simulink model "alfa147gta"  (R2013a)
settings: Solver=ode45  StartTime=0.0  StopTime=10.0  RelTol=1e-3
PreLoadFcn:
  | load('alfa147gta.mat')
undefined symbols (not defined in the file): EngineRPM, EngineTRQ, FinalRatio, GearRatio, Kdrag, Mass, WheelRadius
settings Model: Creator=luca  LastModifiedBy=luca

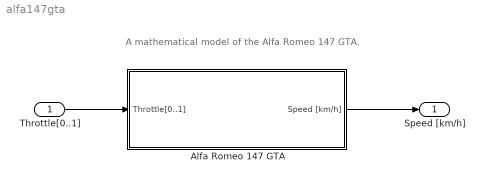
== system alfa147gta ==
  note: A mathematical model of the Alfa Romeo 147 GTA.
  Throttle[0..1] : Inport
  Alfa Romeo 147 GTA : Subsystem
  Speed [km/h] : Outport
  wires:
  Throttle[0..1]/1 -> Alfa Romeo 147 GTA/1(Throttle[0..1])
  Alfa Romeo 147 GTA/1(Speed [km/h]) -> Speed [km/h]/1

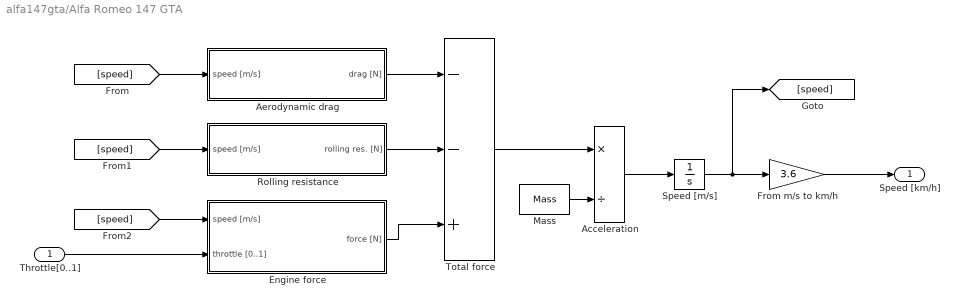
== system alfa147gta/Alfa Romeo 147 GTA ==
  Throttle[0..1] : Inport
  Acceleration : Product  Inputs=*/
  Aerodynamic drag : Subsystem
  Engine force : Subsystem
  From m/s to km/h : Gain  Gain=3.6
  Mass : Constant  Value=Mass
  Rolling resistance : Subsystem
  Speed [m/s] : Integrator
  Total force : Sum  Inputs=--+
  Speed [km/h] : Outport
  wires:
  Engine force/1(force [N]) -> Total force/3
  Rolling resistance/1(rolling res. [N]) -> Total force/2
  Aerodynamic drag/1(drag [N]) -> Total force/1
  Total force/1 -> Acceleration/1
  Mass/1 -> Acceleration/2
  Acceleration/1 -> Speed [m/s]/1
  Speed [m/s]/1 -> [speed], From m/s to km/h/1
  From m/s to km/h/1 -> Speed [km/h]/1
  [speed] -> Aerodynamic drag/1(speed [m/s])
  [speed] -> Rolling resistance/1(speed [m/s])
  Throttle[0..1]/1 -> Engine force/2(throttle [0..1])
  [speed] -> Engine force/1(speed [m/s])

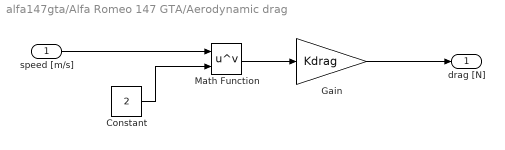
== system alfa147gta/Alfa Romeo 147 GTA/Aerodynamic drag ==
  speed [m/s] : Inport
  Constant : Constant  Value=2
  Gain : Gain  Gain=Kdrag
  Math Function : Math  Operator=pow  SaturateOnIntegerOverflow=on
  drag [N] : Outport
  wires:
  speed [m/s]/1 -> Math Function/1
  Constant/1 -> Math Function/2
  Math Function/1 -> Gain/1
  Gain/1 -> drag [N]/1

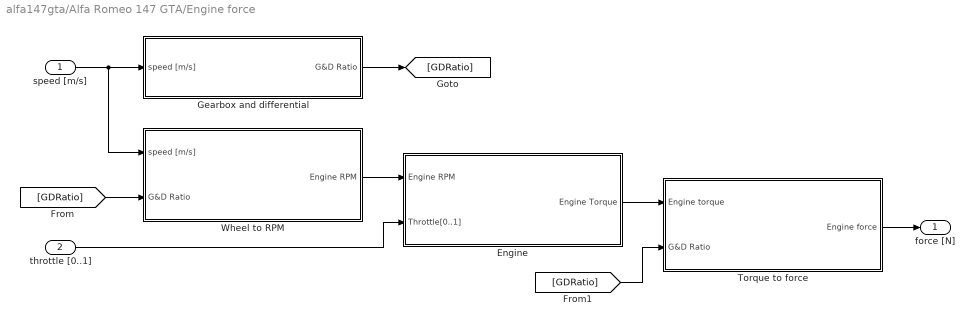
== system alfa147gta/Alfa Romeo 147 GTA/Engine force ==
  speed [m/s] : Inport
  throttle [0..1] : Inport  Port=2
  Engine : Subsystem
  Gearbox and differential : Subsystem
  Torque to force : Subsystem
  Wheel to RPM : Subsystem
  force [N] : Outport
  wires:
  Wheel to RPM/1(Engine RPM) -> Engine/1(Engine RPM)
  throttle [0..1]/1 -> Engine/2(Throttle[0..1])
  speed [m/s]/1 -> Gearbox and differential/1(speed [m/s]), Wheel to RPM/1(speed [m/s])
  Engine/1(Engine Torque) -> Torque to force/1(Engine torque)
  Torque to force/1(Engine force) -> force [N]/1
  Gearbox and differential/1(G&D Ratio) -> [GDRatio]
  [GDRatio] -> Wheel to RPM/2(G&D Ratio)
  [GDRatio] -> Torque to force/2(G&D Ratio)

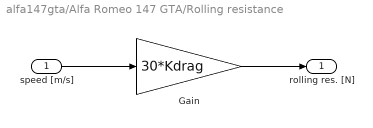
== system alfa147gta/Alfa Romeo 147 GTA/Rolling resistance ==
  speed [m/s] : Inport
  Gain : Gain  Gain=30*Kdrag
  rolling res. [N] : Outport
  wires:
  speed [m/s]/1 -> Gain/1
  Gain/1 -> rolling res. [N]/1

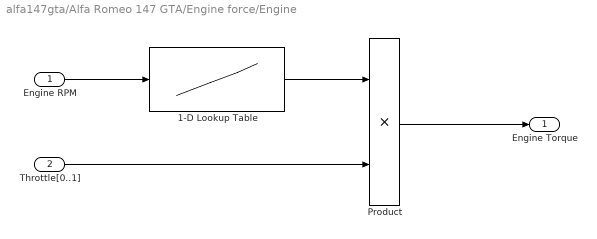
== system alfa147gta/Alfa Romeo 147 GTA/Engine force/Engine ==
  Engine RPM : Inport
  Throttle[0..1] : Inport  Port=2
  1-D Lookup Table : Lookup_n-D  NumberOfTableDimensions=1  BreakpointsForDimension1=EngineRPM  Table=EngineTRQ  InterpMethod=Cubic spline  RndMeth=Simplest  InputSameDT=on
  Product : Product
  Engine Torque : Outport
  wires:
  Engine RPM/1 -> 1-D Lookup Table/1
  Throttle[0..1]/1 -> Product/2
  1-D Lookup Table/1 -> Product/1
  Product/1 -> Engine Torque/1

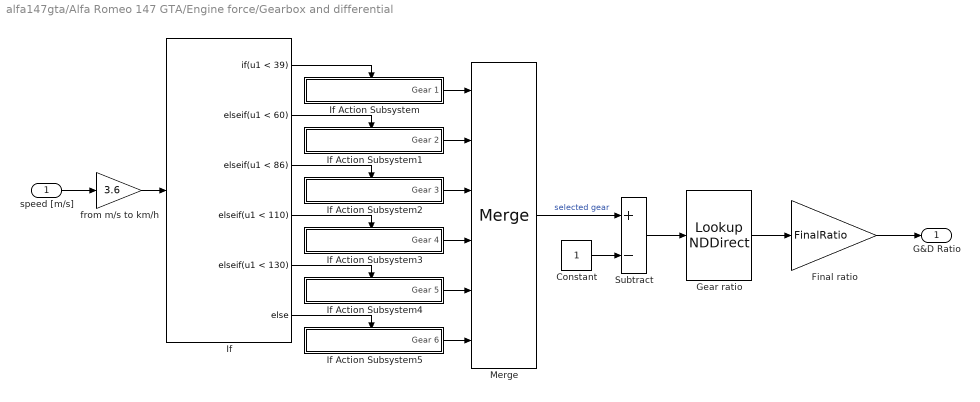
== system alfa147gta/Alfa Romeo 147 GTA/Engine force/Gearbox and differential ==
  speed [m/s] : Inport
  Constant : Constant
  Final ratio : Gain  Gain=FinalRatio
  Gear ratio : LookupNDDirect  NumberOfTableDimensions=1  Table=GearRatio
  If : If  IfExpression=u1 < 39  ElseIfExpressions=u1 < 60, u1 < 86, u1 < 110, u1 < 130
  If Action Subsystem : Subsystem  TreatAsAtomicUnit=on
  If Action Subsystem1 : Subsystem  TreatAsAtomicUnit=on
  If Action Subsystem2 : Subsystem  TreatAsAtomicUnit=on
  If Action Subsystem3 : Subsystem  TreatAsAtomicUnit=on
  If Action Subsystem4 : Subsystem  TreatAsAtomicUnit=on
  If Action Subsystem5 : Subsystem  TreatAsAtomicUnit=on
  Merge : Merge  Inputs=6
  Subtract : Sum  Inputs=+-
  from m/s to km/h : Gain  Gain=3.6
  G&D Ratio : Outport
  wires:
  speed [m/s]/1 -> from m/s to km/h/1
  from m/s to km/h/1 -> If/1
  If/1 -> If Action Subsystem/Action
  If/2 -> If Action Subsystem1/Action
  If/3 -> If Action Subsystem2/Action
  If/4 -> If Action Subsystem3/Action
  If/5 -> If Action Subsystem4/Action
  If/6 -> If Action Subsystem5/Action
  If Action Subsystem/1(Gear 1) -> Merge/1
  If Action Subsystem1/1(Gear 2) -> Merge/2
  If Action Subsystem2/1(Gear 3) -> Merge/3
  If Action Subsystem3/1(Gear 4) -> Merge/4
  If Action Subsystem4/1(Gear 5) -> Merge/5
  If Action Subsystem5/1(Gear 6) -> Merge/6
  Gear ratio/1 -> Final ratio/1
  Final ratio/1 -> G&D Ratio/1
  Merge/1 -> Subtract/1  "selected gear"
  Subtract/1 -> Gear ratio/1
  Constant/1 -> Subtract/2

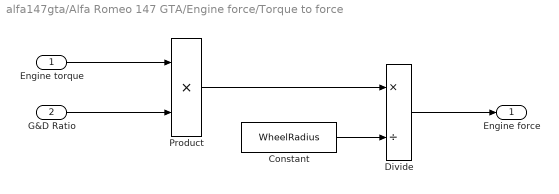
== system alfa147gta/Alfa Romeo 147 GTA/Engine force/Torque to force ==
  Engine torque : Inport
  G&D Ratio : Inport  Port=2
  Constant : Constant  Value=WheelRadius
  Divide : Product  Inputs=*/
  Product : Product
  Engine force : Outport
  wires:
  Engine torque/1 -> Product/1
  G&D Ratio/1 -> Product/2
  Product/1 -> Divide/1
  Constant/1 -> Divide/2
  Divide/1 -> Engine force/1

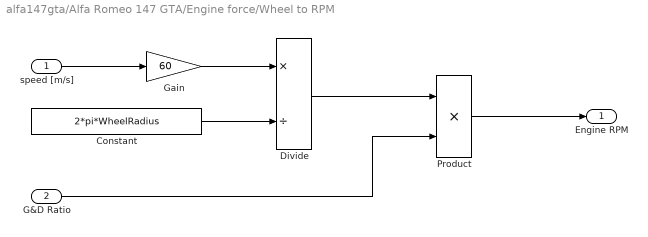
== system alfa147gta/Alfa Romeo 147 GTA/Engine force/Wheel to RPM ==
  speed [m/s] : Inport
  G&D Ratio : Inport  Port=2
  Constant : Constant  Value=2*pi*WheelRadius
  Divide : Product  Inputs=*/
  Gain : Gain  Gain=60
  Product : Product
  Engine RPM : Outport
  wires:
  speed [m/s]/1 -> Gain/1
  Gain/1 -> Divide/1
  Constant/1 -> Divide/2
  Divide/1 -> Product/1
  G&D Ratio/1 -> Product/2
  Product/1 -> Engine RPM/1

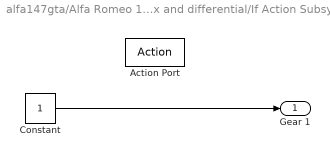
== system alfa147gta/Alfa Romeo 147 GTA/Engine force/Gearbox and differential/If Action Subsystem ==
  Action Port : ActionPort  ActionType=then
  Constant : Constant
  Gear 1 : Outport  InitialOutput=1
  wires:
  Constant/1 -> Gear 1/1

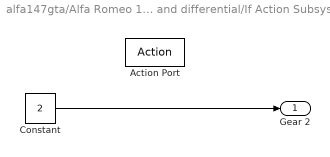
== system alfa147gta/Alfa Romeo 147 GTA/Engine force/Gearbox and differential/If Action Subsystem1 ==
  Action Port : ActionPort  ActionType=elseif
  Constant : Constant  Value=2
  Gear 2 : Outport  InitialOutput=2
  wires:
  Constant/1 -> Gear 2/1

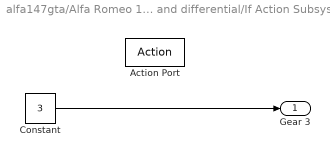
== system alfa147gta/Alfa Romeo 147 GTA/Engine force/Gearbox and differential/If Action Subsystem2 ==
  Action Port : ActionPort  ActionType=elseif
  Constant : Constant  Value=3
  Gear 3 : Outport  InitialOutput=3
  wires:
  Constant/1 -> Gear 3/1

== system alfa147gta/Alfa Romeo 147 GTA/Engine force/Gearbox and differential/If Action Subsystem3 ==
  Action Port : ActionPort  ActionType=elseif
  Constant : Constant  Value=4
  Gear 4 : Outport  InitialOutput=4
  wires:
  Constant/1 -> Gear 4/1

== system alfa147gta/Alfa Romeo 147 GTA/Engine force/Gearbox and differential/If Action Subsystem4 ==
  Action Port : ActionPort  ActionType=elseif
  Constant : Constant  Value=5
  Gear 5 : Outport  InitialOutput=5
  wires:
  Constant/1 -> Gear 5/1

== system alfa147gta/Alfa Romeo 147 GTA/Engine force/Gearbox and differential/If Action Subsystem5 ==
  Action Port : ActionPort  ActionType=else
  Constant : Constant  Value=6
  Gear 6 : Outport  InitialOutput=6
  wires:
  Constant/1 -> Gear 6/1
